simulink model "CruiseControl_RP_reqCheck_harness"  (R2015a)
settings: Solver=FixedStepDiscrete  StartTime=0.0  StopTime=inf  FixedStep=0.1  RelTol=1e-3
PreLoadFcn:
  | CruiseControl_dd_RP;
model workspace (MAT data in the model file):
  min_throttle = 0.6
  min_speed = 20
undefined symbols (not defined in the file or in its folder): maxtspeed, mintspeed
settings Model: SldvGeneratedHarnessModel=TestUnitModel=CruiseControl_RP|  CovMetricSettings=dcme  CovHTMLOptions=-sRT=0 -sVT=0 -aTS=1 -bRG=1 -bTC=0 -hTR=0 -nFC=0 -scm=1 -bcm=1 -xEv=0  CovHtmlReporting=off  CovSaveSingleToWorkspaceVar=off  CovCumulativeReport=on  CovModelRefEnable=all  CovSFcnEnable=off  Creator=The MathWorks Inc.  LastModifiedBy=colosky
settings DataIOCC: SaveFormat=StructureWithTime  SaveOutput=off  SaveTime=off
settings OptimizationCC: ExpressionDepthLimit=2147483647  InitFltsAndDblsToZero=on  OptimizeModelRefInitCode=on
settings DebuggingCC: SaveWithParameterizedLinksMsg=none  UnderspecifiedInitializationDetection=Classic  MergeDetectMultiDrivingBlocksExec=none  SolverPrmCheckMsg=warning  InheritedTsInSrcMsg=none  FcnCallInpInsideContextMsg=UseLocalSettings  StateNameClashWarn=warning  StrictBusMsg=ErrorOnBusTreatedAsVector
settings ModelReferenceCC: ModelReferenceNumInstancesAllowed=Single
settings SFSimCC: SimParseCustomCode=off
settings RTWCC: SystemTargetFile=ert.tlc  TemplateMakefile=ert_default_tmf  Description=Embedded Coder  GenerateReport=on  IncludeHyperlinkInReport=on  LaunchReport=on  PortableWordSizes=on  GenerateTraceInfo=on  GenerateTraceReport=on  GenerateTraceReportSl=on  GenerateTraceReportSf=on  GenerateTraceReportEml=on  GenerateWebview=on
settings CodeAppCC: IgnoreCustomStorageClasses=off
settings ERTTargetCC: ParMdlRefBuildCompliant=on  CompOptLevelCompliant=on  ConcurrentExecutionCompliant=on  ERTFirstTimeCompliant=on  SupportContinuousTime=off  SupportVariableSizeSignals=off  ModelStepFunctionPrototypeControlCompliant=on  CPPClassGenCompliant=on  InlinedParameterPlacement=Hierarchical  ERTCustomFileTemplate=example_file_process.tlc
settings ConfigComp: Description=Design Verifier Custom Configuration Component  DVMode=DesignErrorDetection  DVMaxProcessTime=3000  DVDisplayUnsatisfiableObjectives=on  DVAutomaticStubbing=off  DVMakeOutputFilesUnique=off  DVParametersConfigFileName=NV_Cruise_new_sldv_params.m  DVModelCoverageObjectives=MCDC  DVMaxTestCaseSteps=500  DVTestSuiteOptimization=CombinedObjectives  DVAssertions=EnableAll  DVProofAssumptions=EnableAll  DVIgnoreCovSatisfied=on  DVCoverageDataFile=CruiseControlCovManual.cvt  DVDetectIntegerOverflow=off  DVDetectDeadLogic=on  DVDetectActiveLogic=on  DVMaxViolationSteps=50  DVSaveDataFile=off  DVReportIncludeGraphics=on

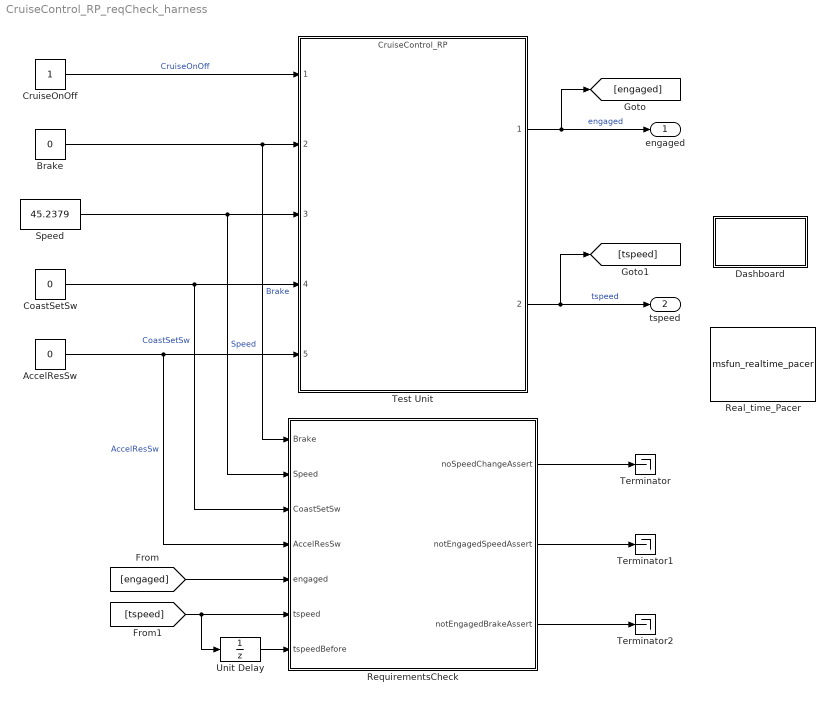
== system CruiseControl_RP_reqCheck_harness ==
  AccelResSw : Constant  Value=0  OutDataTypeStr=boolean
      settings: OpenFcn=|
      | val = ~str2num(get_param(gcb,'Value'));
      | set_param(gcb,'Value',num2str(val));
      | if val
      |    set_param(gcb,'BackgroundColor','green');
      | else
      |    set_param(gcb,'BackgroundColor','red');
      | end
  Brake : Constant  Value=0  OutDataTypeStr=boolean
      settings: OpenFcn=|
      | val = ~str2num(get_param(gcb,'Value'));
      | set_param(gcb,'Value',num2str(val));
      | if val
      |    set_param(gcb,'BackgroundColor','green');
      | else
      |    set_param(gcb,'BackgroundColor','red');
      | end
  CoastSetSw : Constant  Value=0  OutDataTypeStr=boolean
      settings: OpenFcn=|
      | val = ~str2num(get_param(gcb,'Value'));
      | set_param(gcb,'Value',num2str(val));
      | if val
      |    set_param(gcb,'BackgroundColor','green');
      | else
      |    set_param(gcb,'BackgroundColor','red');
      | end
  CruiseOnOff : Constant  OutDataTypeStr=boolean
      settings: OpenFcn=|
      | val = ~str2num(get_param(gcb,'Value'));
      | set_param(gcb,'Value',num2str(val));
      | if val
      |    set_param(gcb,'BackgroundColor','green');
      | else
      |    set_param(gcb,'BackgroundColor','red');
      | end
  Dashboard : Subsystem
      mask Display: disp('Dashboard');
  Real_time_Pacer : M-S-Function  FunctionName=msfun_realtime_pacer  Parameters=realTimeScaleFactor, overRunOutputEnable  mask(Real-time Pacer){realTimeOne=on, overRunOutput=off, realTimeScaleFactor=1, overRunOutputEnable=0}
      mask prompts: realTimeOne "Real-time"; overRunOutput "Output Over-run Indicator"; realTimeScaleFactor "Scaled Real-time Factor (sim sec/clock sec)"
      mask help:
      | 1)  Check "Real-time" to run the model at a real-time pace.
      | 2)  Or uncheck "Real-time" to run the model at a scaled real-time pace (sim sec/clock sec)
      mask init:
      | if strcmp(get_param(gcb,'overRunOutput'),'on')
      |      set_param(gcb,'overRunOutputEnable','1');
      |      overRunOutputEnable = 1;
      | else
      |      set_param(gcb,'overRunOutputEnable','0');
      |      overRunOutputEnable = 0;
      | end
      mask Callback realTimeOne:
      | if strcmp(get_param(gcb,'realTimeOne'),'on')
      |     set_param(gcb,'MaskEnables',{'on' 'on' 'off' 'off'});
      |     set_param(gcb,'realTimeScaleFactor','1');
      | else
      |     set_param(gcb,'MaskEnables',{'on' 'on' 'on' 'off'})
      | end
      mask DialogControl ParameterGroupVar Prompt: Real-time Pacer Settings
      mask Display:
      | % port_label('output', 1, 'overRun');
      | disp(['Real-time' char(10) char(10) 'Pacer']);
  RequirementsCheck : MATLAB Function  TreatAsAtomicUnit=on
  Speed : Constant  Value=45.2379  OutMin=0  OutMax=120  OutDataTypeStr=Inherit: Inherit via back propagation
  Terminator : Terminator
  Terminator1 : Terminator
  Terminator2 : Terminator
  Test Unit : ModelReference  ModelNameDialog=CruiseControl_RP  SimulationMode=Normal  ModelReferenceVersion=1.327  CopyOfModelName=CruiseControl_RP
  Unit Delay : UnitDelay  SampleTime=-1
  engaged : Outport
  tspeed : Outport  Port=2
  wires:
  CruiseOnOff/1 -> Test Unit/1  "CruiseOnOff"
  Brake/1 -> RequirementsCheck/1(Brake), Test Unit/2  "Brake"
  Speed/1 -> RequirementsCheck/2(Speed), Test Unit/3  "Speed"
  CoastSetSw/1 -> RequirementsCheck/3(CoastSetSw), Test Unit/4  "CoastSetSw"
  AccelResSw/1 -> RequirementsCheck/4(AccelResSw), Test Unit/5  "AccelResSw"
  Test Unit/1 -> [engaged], engaged/1  "engaged"
  Test Unit/2 -> [tspeed], tspeed/1  "tspeed"
  [engaged] -> RequirementsCheck/5(engaged)
  [tspeed] -> Unit Delay/1, RequirementsCheck/6(tspeed)
  Unit Delay/1 -> RequirementsCheck/7(tspeedBefore)
  RequirementsCheck/1(noSpeedChangeAssert) -> Terminator/1
  RequirementsCheck/2(notEngagedSpeedAssert) -> Terminator1/1
  RequirementsCheck/3(notEngagedBrakeAssert) -> Terminator2/1

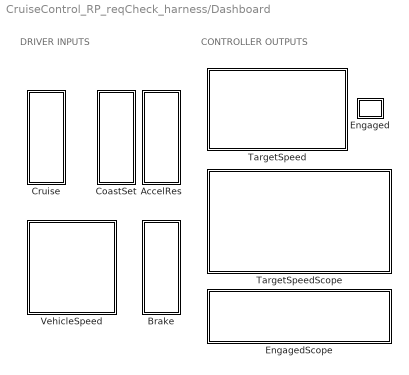
== system CruiseControl_RP_reqCheck_harness/Dashboard ==
  note: CONTROLLER OUTPUTS
  note: DRIVER INPUTS
  AccelRes : Subsystem  DialogController=hmiCreateDDGDialog  IsWebBlock=on  mask(MathWorksWebBlock){webBlockId=5f61b1b7-d845-4c9e-a44e-ef817fa1dfea, webBlockType=rockerswitch, ShowInLibBrowser=on, ShowInitialText=on, HMISrcModelName=CruiseControl_RP_level_harness}
      mask prompts: webBlockId "WebBlock Id"; webBlockType "WebBlock Type"; HMISrcModelName "Source Model"
      mask Help: helpview([docroot '/mapfiles/simulink.map'], 'hmi_rocker_switch')
      mask Display:
      | if strcmp(get_param(bdroot(gcb),'BlockDiagramType'), 'library')
      |     image([(matlabroot) '/toolbox/simulink/hmi/icons/RockerSwitch.png']);
      | end
  Brake : Subsystem  DialogController=hmiCreateDDGDialog  IsWebBlock=on  mask(MathWorksWebBlock){webBlockId=4e900736-6a9d-4f5c-adc3-6bdf00d7cb23, webBlockType=rockerswitch, ShowInLibBrowser=on, ShowInitialText=on, HMISrcModelName=CruiseControl_RP_level_harness}
      mask prompts: webBlockId "WebBlock Id"; webBlockType "WebBlock Type"; HMISrcModelName "Source Model"
      mask Help: helpview([docroot '/mapfiles/simulink.map'], 'hmi_rocker_switch')
      mask Display:
      | if strcmp(get_param(bdroot(gcb),'BlockDiagramType'), 'library')
      |     image([(matlabroot) '/toolbox/simulink/hmi/icons/RockerSwitch.png']);
      | end
  CoastSet : Subsystem  DialogController=hmiCreateDDGDialog  IsWebBlock=on  mask(MathWorksWebBlock){webBlockId=9d1e2fa4-8365-4be6-9381-b66520279f19, webBlockType=rockerswitch, ShowInLibBrowser=on, ShowInitialText=on, HMISrcModelName=CruiseControl_RP_level_harness}
      mask prompts: webBlockId "WebBlock Id"; webBlockType "WebBlock Type"; HMISrcModelName "Source Model"
      mask Help: helpview([docroot '/mapfiles/simulink.map'], 'hmi_rocker_switch')
      mask Display:
      | if strcmp(get_param(bdroot(gcb),'BlockDiagramType'), 'library')
      |     image([(matlabroot) '/toolbox/simulink/hmi/icons/RockerSwitch.png']);
      | end
  Cruise : Subsystem  DialogController=hmiCreateDDGDialog  IsWebBlock=on  mask(MathWorksWebBlock){webBlockId=a8253440-ca89-4c37-8285-ad16728eeda2, webBlockType=rockerswitch, ShowInLibBrowser=on, ShowInitialText=on, HMISrcModelName=CruiseControl_RP_level_harness}
      mask prompts: webBlockId "WebBlock Id"; webBlockType "WebBlock Type"; HMISrcModelName "Source Model"
      mask Help: helpview([docroot '/mapfiles/simulink.map'], 'hmi_rocker_switch')
      mask Display:
      | if strcmp(get_param(bdroot(gcb),'BlockDiagramType'), 'library')
      |     image([(matlabroot) '/toolbox/simulink/hmi/icons/RockerSwitch.png']);
      | end
  Engaged : Subsystem  DialogController=hmiCreateDDGDialog  IsWebBlock=on  mask(MathWorksWebBlock){webBlockId=5364136f-78d0-48a5-a0e8-c7a5285a8b05, webBlockType=lamp, ShowInLibBrowser=on, ShowInitialText=on, HMISrcModelName=CruiseControl_RP_level_harness}
      mask prompts: webBlockType "WebBlock Type"; HMISrcModelName "Source Model"
      mask Help: helpview([docroot '/mapfiles/simulink.map'], 'hmi_lamp')
      mask Display:
      | if strcmp(get_param(bdroot(gcb),'BlockDiagramType'), 'library')
      |     image([(matlabroot) '/toolbox/simulink/hmi/icons/Lamp.png']);
      | end
  EngagedScope : Subsystem  DialogController=hmiCreateDDGDialog  IsWebBlock=on  mask(MathWorksWebBlock){webBlockId=21b9a1b7-b9bb-41cb-8ef1-a1f0edbd3ff7, webBlockType=sdiscope, ShowInitialText=on, HMISrcModelName=CruiseControl_RP_level_harness}
      mask prompts: webBlockId "WebBlock Id"; webBlockType "WebBlock Type"; HMISrcModelName "Source Model"
      mask Help: helpview([docroot '/mapfiles/simulink.map'], 'hmi_scope')
      mask Display:
      | if strcmp(get_param(bdroot(gcb),'BlockDiagramType'), 'library')
      |     image([(matlabroot) '/toolbox/simulink/hmi/icons/DashboardScope.png']);
      | end
  TargetSpeed : Subsystem  DialogController=hmiCreateDDGDialog  IsWebBlock=on  mask(MathWorksWebBlock){webBlockId=da626fbd-e858-42ae-a6d0-5e16f4b084cd, webBlockType=semicirculargauge, ShowInLibBrowser=on, ShowInitialText=on, HMISrcModelName=CruiseControl_RP_level_harness}
      mask prompts: webBlockId "WebBlock Id"; webBlockType "WebBlock Type"; HMISrcModelName "Source Model"
      mask Help: helpview([docroot '/mapfiles/simulink.map'], 'hmi_half_gauge')
      mask Display:
      | if strcmp(get_param(bdroot(gcb),'BlockDiagramType'), 'library')
      |     image([(matlabroot) '/toolbox/simulink/hmi/icons/SemicircularGauge.png']);
      | end
  TargetSpeedScope : Subsystem  DialogController=hmiCreateDDGDialog  IsWebBlock=on  mask(MathWorksWebBlock){webBlockId=14557e63-52d1-44de-9e22-324a19bc6f41, webBlockType=sdiscope, ShowInitialText=on, HMISrcModelName=CruiseControl_RP_level_harness}
      mask prompts: webBlockId "WebBlock Id"; webBlockType "WebBlock Type"; HMISrcModelName "Source Model"
      mask Help: helpview([docroot '/mapfiles/simulink.map'], 'hmi_scope')
      mask Display:
      | if strcmp(get_param(bdroot(gcb),'BlockDiagramType'), 'library')
      |     image([(matlabroot) '/toolbox/simulink/hmi/icons/DashboardScope.png']);
      | end
  VehicleSpeed : Subsystem  DialogController=hmiCreateDDGDialog  IsWebBlock=on  mask(MathWorksWebBlock){webBlockId=31446eca-20b6-47c8-beed-79f89e0abe36, webBlockType=continuousknob, ShowInLibBrowser=on, ShowInitialText=on, HMISrcModelName=CruiseControl_RP_level_harness}
      mask prompts: webBlockId "WebBlock Id"; webBlockType "WebBlock Type"; HMISrcModelName "Source Model"
      mask Help: helpview([docroot '/mapfiles/simulink.map'], 'hmi_knob')
      mask Display:
      | if strcmp(get_param(bdroot(gcb),'BlockDiagramType'), 'library')
      |     image([(matlabroot) '/toolbox/simulink/hmi/icons/ContinuousKnob.png']);
      | end

== system CruiseControl_RP_reqCheck_harness/Dashboard/AccelRes ==

== system CruiseControl_RP_reqCheck_harness/Dashboard/Brake ==

== system CruiseControl_RP_reqCheck_harness/Dashboard/CoastSet ==

== system CruiseControl_RP_reqCheck_harness/Dashboard/Cruise ==

== system CruiseControl_RP_reqCheck_harness/Dashboard/Engaged ==

== system CruiseControl_RP_reqCheck_harness/Dashboard/EngagedScope ==

== system CruiseControl_RP_reqCheck_harness/Dashboard/TargetSpeed ==

== system CruiseControl_RP_reqCheck_harness/Dashboard/TargetSpeedScope ==

== system CruiseControl_RP_reqCheck_harness/Dashboard/VehicleSpeed ==

== matlab function CruiseControl_RP_reqCheck_harness/RequirementsCheck ==
  data: Brake input; noSpeedChangeAssert output; Speed input; CoastSetSw input; AccelResSw input; engaged input; tspeed input; tspeedBefore input; notEngagedSpeedAssert output; notEngagedBrakeAssert output; maxtspeed parameter; mintspeed parameter
function [noSpeedChangeAssert, notEngagedSpeedAssert, notEngagedBrakeAssert] ...
    = RequirementsCheck(Brake, Speed, CoastSetSw, AccelResSw, ...
    engaged, tspeed, tspeedBefore, maxtspeed, mintspeed)
    
    % init Asserts
    noSpeedChangeAssert = true;
    notEngagedSpeedAssert = true;
    notEngagedBrakeAssert = true;

    % check Asserts    
    if (~AccelResSw && ~CoastSetSw)
        % noSpeedChange
        noSpeedChangeAssert = (tspeed==tspeedBefore);

    elseif (Speed>maxtspeed || Speed<mintspeed)
        % notEngagedSpeedLimit
        notEngagedSpeedAssert = ~engaged;

    elseif Brake
        % notEngagedBraking
        notEngagedBrakeAssert = ~engaged;
    end

end
